simulink model "sin1000FFT"  (Simulink 7.0)
settings: Solver=ode45  StartTime=0.0  StopTime=0.1  RelTol=1e-3
undefined symbols (not defined in the file or in its folder): get
libraries: dspsnks4 x2, dspwin32 x1, dspbuff3 x1
settings Model: Creator=ouassarni  LastModifiedBy=ouassarni

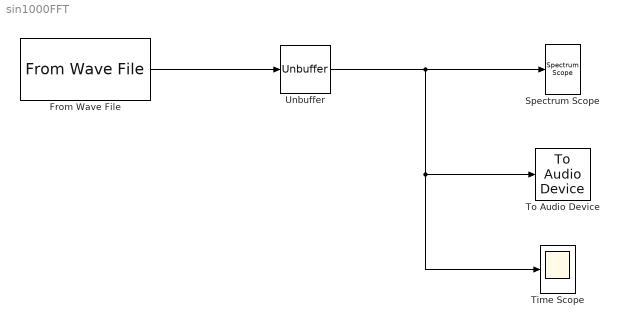
== system sin1000FFT ==
  From Wave File : dspwin32/From Wave File  FileName=sin1000.wav  SamplesPerFrame=256  MinBufSize=256  dType=double  bLoop=off  timesToPlay=1  restartMode=immediately after last sample  firstSampleOutput=off  lastSampleOutput=off
  Spectrum Scope : dspsnks4/Spectrum Scope  DialogController=dspdialog.SpectrumScope  DialogControllerArgs=DataTag0  SystemSampleTime=-1  ScopeProperties=on  Domain=Frequency  HorizSpan=1  UseBuffer=on  BufferSize=128  Overlap=64  inpFftLenInherit=off  FFTlength=128  numAvg=2  DisplayProperties=off  AxisGrid=on  Memory=off  FrameNumber=on  AxisLegend=off  AxisZoom=off  OpenScopeAtSimStart=on  OpenScopeImmediately=off  FigPos=get(0,'defaultfigureposition')  AxisProperties=off  XUnits=Hertz  XRange=[0...Fs/2]  InheritXIncr=on  XIncr=1.0  XLabel=Samples  XLimit=Auto  YUnits=dB  XMax=1  XMin=0  YLabel=Magnitude-squared, dB  LineProperties=off  wintypeSpecScope=Hann  RsSpecScope=50  betaSpecScope=5  winsampSpecScope=Periodic
      settings: YMin=-0  YMax=20
  Time Scope : Scope
      settings: DataFormat=Structure
  To Audio Device : dspsnks4/To Audio Device  DialogController=dspDDGCreate  DialogControllerArgs=DataTag1  deviceName=Default  inheritSampleRate=on  sampleRate=44100  deviceDatatype=Determine from input data type  autoBufferSize=on  bufferSize=4096  queueDuration=1.0
  Unbuffer : dspbuff3/Unbuffer  ic=0
  wires:
  Unbuffer/1 -> Spectrum Scope/1, Time Scope/1, To Audio Device/1
  From Wave File/1 -> Unbuffer/1
